simulink model "chamberPortSim"  (R2020b)
settings: Solver=VariableStepAuto  StartTime=0.0  StopTime=10.0  RelTol=1e-3
undefined symbols (not defined in the file or in its folder): Sim
settings Model: Creator=Edward  LastModifiedBy=Edward

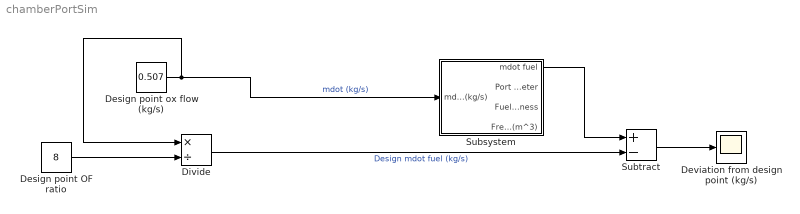
== system chamberPortSim ==
  Design point OF ratio : Constant  Value=8
  Design point ox flow (kg/s) : Constant  Value=0.507
  Deviation from design point (kg/s) : Scope
  Divide : Product  Inputs=*/
  Subsystem : Subsystem  mask{useOxidiserFluxOnlyRegRateEquation=Sim.combustionChamber.useOxFluxRegRateEquation}
      mask prompts: useOxidiserFluxOnlyRegRateEquation "Use oxidiser flux only reg rate model?"
  Subtract : Sum  Inputs=+-
  wires:
  Design point ox flow (kg/s)/1 -> Subsystem/1(mdot (kg/s)), Divide/1  "mdot (kg/s)"
  Design point OF ratio/1 -> Divide/2
  Divide/1 -> Subtract/2  "Design mdot fuel (kg/s)"
  Subtract/1 -> Deviation from design point (kg/s)/1
  Subsystem/1(mdot fuel) -> Subtract/1

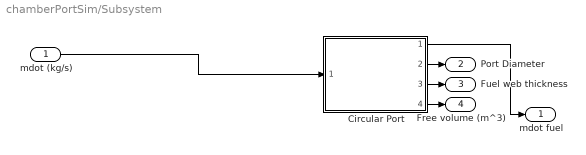
== system chamberPortSim/Subsystem ==
  mdot (kg/s) : Inport
  Circular Port : Subsystem  ReferencedSubsystem=Circular_Port_Model
  mdot fuel : Outport
  Port Diameter : Outport  Port=2
  Fuel web thickness : Outport  Port=3
  Free volume (m^3) : Outport  Port=4
  wires:
  Circular Port/1 -> mdot fuel/1
  mdot (kg/s)/1 -> Circular Port/1
  Circular Port/4 -> Free volume (m^3)/1
  Circular Port/3 -> Fuel web thickness/1
  Circular Port/2 -> Port Diameter/1
